simulink model "example"  (R2025a)
settings: Solver=FixedStepAuto  StartTime=0.0  StopTime=15  RelTol=1e-3  EnableMultiTasking=on
undefined symbols (not defined in the file): f
libraries: simulink x3, aerolibfltsims x2, instrumentlib x2, aerolibobsolete x1, aerolibconvert2 x1
Description:
  | Simulink(R) 3D Animation(TM) - Tutorial #2
  | 
  | This model represents a tutorial example described in the documentation. See the 'Associate
  | Virtual Worlds with Simulink' chapter in the Simulink 3D Animation User's Guide.
settings Model: ExtModeTrigMode=oneshot  ExtModeArmWhenConnect=off  Creator=The MathWorks, Inc.  LastModifiedBy=Ethan Phillips
settings SolverCC: AlgebraicLoopSolver=TrustRegion  AutoInsertRateTranBlk=on
settings DataIOCC: LimitDataPoints=on  SaveFormat=Array  SaveOutput=off  SaveTime=off  ReturnWorkspaceOutputs=off  SignalLoggingName=logsOut
settings OptimizationCC: BlockReduction=off  BooleanDataType=off  ExpressionDepthLimit=2147483647.0  InitFltsAndDblsToZero=on  LifeSpan=inf
settings DebuggingCC: UnderspecifiedInitializationDetection=Classic  MergeDetectMultiDrivingBlocksExec=none  CheckExecutionContextPreStartOutputMsg=on  SignalResolutionControl=TryResolveAllWithWarning  MultiTaskDSMMsg=warning  MultiTaskCondExecSysMsg=none  FcnCallInpInsideContextMsg=warning  UnconnectedInputMsg=warning  UnconnectedOutputMsg=warning  UnconnectedLineMsg=warning  StateNameClashWarn=warning  SymbolicDimsDataTypeCodeGenerationDiagnostic=none  SFUnexpectedBacktrackingDiag=warning  SFNoUnconditionalDefaultTransitionDiag=warning  SFExecutionAtInitializationDiag=none  ArithmeticOperatorsInVariantConditions=warning
settings HardwareCC: ProdBitPerPointer=32.0  ProdBitPerSizeT=32.0  ProdBitPerPtrDiffT=32.0  ProdLargestAtomicFloat=None  ProdIntDivRoundTo=Undefined  ProdEndianess=Unspecified  ProdWordSize=32.0  ProdHWDeviceType=32-bit Generic  TargetUnknown=on
settings ModelReferenceCC: UpdateModelReferenceTargets=IfOutOfDate  EnableRefExpFcnMdlSchedulingChecks=on  PropagateSignalLabelsOutOfModel=off
settings SFSimCC: SimUseLocalCustomCode=off  CustomCodeUndefinedFunction=UseInterfaceOnly
settings RTWCC: RTWUseLocalCustomCode=off  GPUComputeCapability=3.5
settings CodeAppCC: StateflowObjectComments=on
settings GRTTargetCC: TargetFcnLib=ansi_tfl_tmw.mat  TargetLangStandard=C89/C90 (ANSI)  CombineOutputUpdateFcns=off  GRTInterface=on
settings ConfigComp: CovMetricSettings=d  CovSaveCumulativeToWorkspaceVar=on  CovSaveSingleToWorkspaceVar=on  CovExternalEMLEnable=off  CovSFcnEnable=off

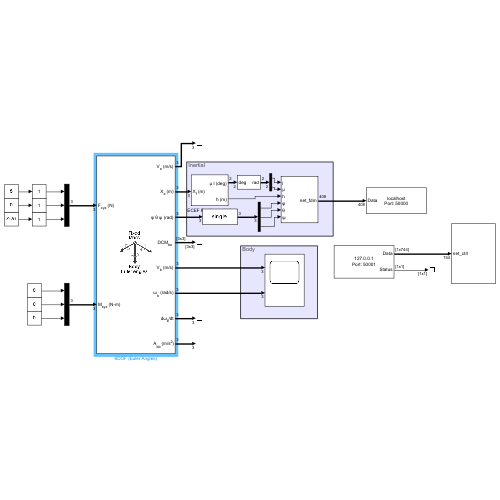
[thumbnail: Simulink's stored preview of the top-level diagram]
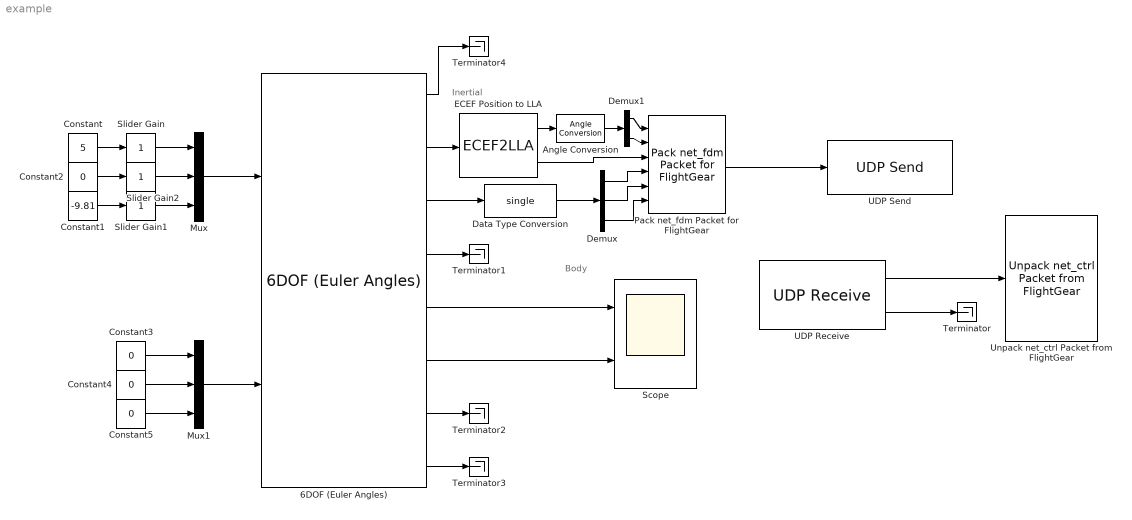
== system example ==
  note: Body
  note: Inertial
  6DOF (Euler Angles) : aerolibobsolete/6DOF (Euler Angles)  units=Metric (MKS)  mtype=Fixed  rep=Euler Angles  xme_0=[3900000, 4902000, -3985500]  Vm_0=[0 1000000 0]  eul_0=[3.14 0 1.56]  pm_0=[0 0 0]  mass_0=1.0  mass_e=0.5  mass_f=2.0  inertia=eye(3)  inertia_e=eye(3)  inertia_f=2*eye(3)  k_quat=1.0  vre_flag=on  abi_flag=off  aMode=0  xme_statename=''  Vm_statename=''  eul_statename=''  quat_statename=''  pm_statename=''  mass_statename=''
  Angle Conversion : aerolibconvert2/Angle Conversion  IU=deg  OU=rad
  Constant : Constant  Value=5
  Constant1 : Constant  Value=-9.81
  Constant{2..5} (4 alike) : Constant  Value=0
  Data Type Conversion : DataTypeConversion  OutDataTypeStr=single  RndMeth=Simplest  SaturateOnIntegerOverflow=off
  Demux : Demux  Outputs=3
  Demux1 : Demux  Outputs=2
  ECEF Position to LLA : ECEF2LLA
  Mux : Mux  Inputs=3
  Mux1 : Mux  Inputs=3
  Pack net_fdm Packet for FlightGear : aerolibfltsims/Pack net_fdm Packet for FlightGear  FlightGearVersion=v2019.1  ShowPositionAttitudeInputs=on  ShowVelocityAccelerationInputs=off  ShowControlSurfacePositionInputs=off  ShowEngineFuelInputs=off  ShowLandingGearInputs=off  ShowEnvironmentInputs=off  SampleTime=1/30  packetVersion=24
  Scope : Scope  NumInputPorts=2
      settings: ActiveDisplayYMinimum=-7.4842430519070433  ActiveDisplayYMaximum=17.665401740524448
  Slider Gain : simulink/Math Operations/Slider Gain  gain=1  low=-1  high=1
  Slider Gain1 : simulink/Math Operations/Slider Gain  gain=1  low=-1  high=1
  Slider Gain2 : simulink/Math Operations/Slider Gain  gain=1  low=-1  high=1
  Terminator{,1..4} (5 alike) : Terminator
  UDP Receive : instrumentlib/UDP Receive  LocalAddress=127.0.0.1  LocalPort=50001  EnablePortSharing=off  Host=localhost  Port=65343  GetLatestData=on  DataSize=[ 1, 744 ]  DataType=uint8  ASCIIFormatting=%f,  Terminator=LF  CustomTerminator=10  ByteOrder=little-endian  EnableBlockingMode=off  Timeout=10  SampleTime=0.2  SimulateUsing=Interpreted execution
  UDP Send : instrumentlib/UDP Send  Host=localhost  Port=50000  LocalAddress=127.0.0.1  LocalPort=-1  EnablePortSharing=on  OutputDatagramPacketSize=4096  ByteOrder=big-endian  EnableBlockingMode=on  SimulateUsing=Interpreted execution
  Unpack net_ctrl Packet from FlightGear : aerolibfltsims/Unpack net_ctrl Packet from FlightGear  FlightGearVersion=v2019.1  ShowControlSurfacePositionOutputs=off  ShowEngineFuelOutputs=off  ShowLandingGearOutputs=off  ShowAvionicOutputs=off  ShowEnvironmentOutputs=off  SampleTime=-1  packetVersion=27
  wires:
  UDP Receive/1 -> Unpack net_ctrl Packet from FlightGear/1
  UDP Receive/2 -> Terminator/1
  6DOF (Euler Angles)/2 -> ECEF Position to LLA/1
  6DOF (Euler Angles)/4 -> Terminator1/1
  6DOF (Euler Angles)/7 -> Terminator2/1
  6DOF (Euler Angles)/8 -> Terminator3/1
  6DOF (Euler Angles)/5 -> Scope/1
  6DOF (Euler Angles)/6 -> Scope/2
  6DOF (Euler Angles)/1 -> Terminator4/1
  6DOF (Euler Angles)/3 -> Data Type Conversion/1
  ECEF Position to LLA/1 -> Angle Conversion/1
  Angle Conversion/1 -> Demux1/1
  Pack net_fdm Packet for FlightGear/1 -> UDP Send/1
  Mux/1 -> 6DOF (Euler Angles)/1
  Slider Gain/1 -> Mux/1
  Constant/1 -> Slider Gain/1
  Constant1/1 -> Slider Gain1/1
  Constant2/1 -> Slider Gain2/1
  Slider Gain2/1 -> Mux/2
  Slider Gain1/1 -> Mux/3
  Constant4/1 -> Mux1/2
  Constant3/1 -> Mux1/1
  Constant5/1 -> Mux1/3
  Mux1/1 -> 6DOF (Euler Angles)/2
  Data Type Conversion/1 -> Demux/1
  Demux1/1 -> Pack net_fdm Packet for FlightGear/1
  Demux1/2 -> Pack net_fdm Packet for FlightGear/2
  ECEF Position to LLA/2 -> Pack net_fdm Packet for FlightGear/3
  Demux/1 -> Pack net_fdm Packet for FlightGear/4
  Demux/2 -> Pack net_fdm Packet for FlightGear/5
  Demux/3 -> Pack net_fdm Packet for FlightGear/6
